simulink model "temp_fahr"  (R2019a)
settings: Solver=VariableStepAuto  StartTime=0.0  StopTime=10.0  RelTol=1e-3
values from neighbouring files (symbols this model uses):
  temp = 8    [TrainingOne.m]
settings Model: Creator=victor  LastModifiedBy=victor

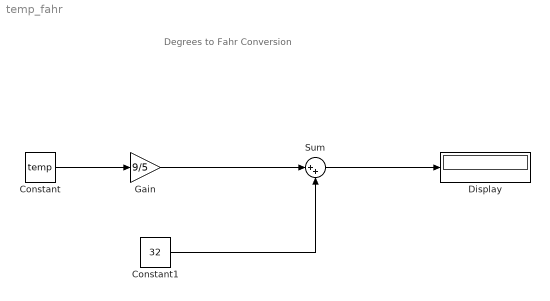
== system temp_fahr ==
  note: Degrees to Fahr Conversion
  Constant : Constant  Value=temp
  Constant1 : Constant  Value=32
  Display : Display
  Gain : Gain  Gain=9/5
  Sum : Sum  Inputs=|++
  wires:
  Constant/1 -> Gain/1
  Gain/1 -> Sum/1
  Constant1/1 -> Sum/2
  Sum/1 -> Display/1
